simulink model "model_with_pursuit"  (R2023b)
settings: Solver=FixedStepAuto  StartTime=0.0  StopTime=10.0  FixedStep=Ts  RelTol=1e-3
values from neighbouring files (symbols this model uses):
  path = path * 0.1    [path_finder_waypoints.m]
  x0 = path(1,1)    [run_pp.m]
  y0 = path(1,2)    [run_pp.m]
undefined symbols (not defined in the file or in its folder): acceleration_limit, alpha, D, dist0, gear, J, Kb, Ki, Ki_turnrate, Kp, Kp_turnrate, Kt, L, M, R, taud, theta0, transport_delay, Ts, turn_acc_limit, wheel_distance, wrad, wzi
libraries: robotalgslib x1
settings Model: Creator=Gianluca  LastModifiedBy=simone

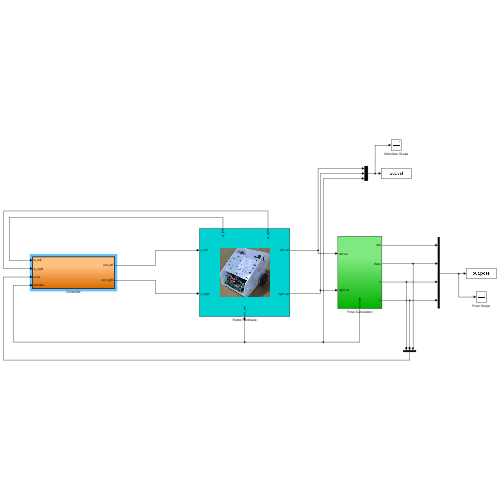
[thumbnail: Simulink's stored preview of the top-level diagram]
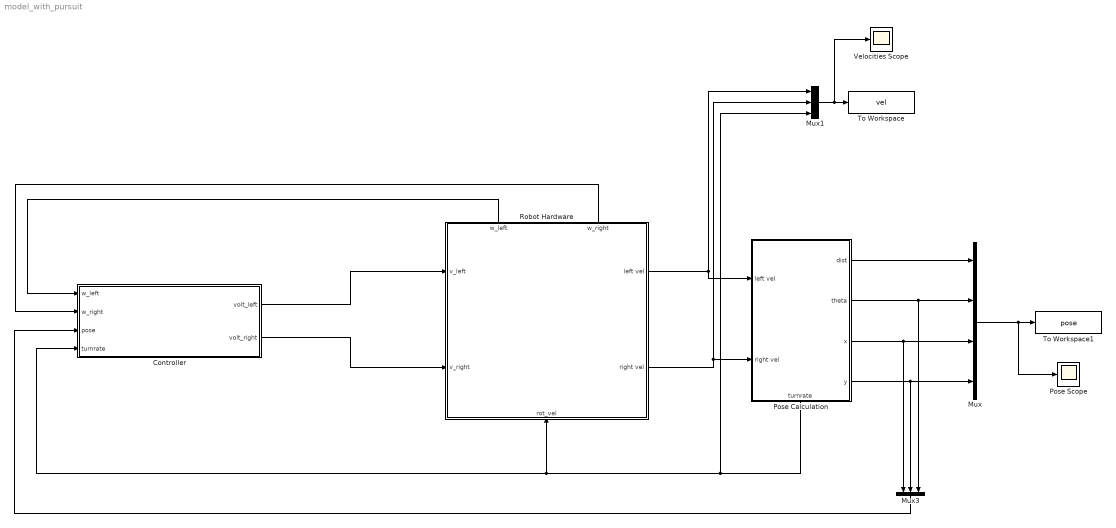
== system model_with_pursuit ==
  Controller : Subsystem  TreatAsAtomicUnit=on
  Mux : Mux
  Mux1 : Mux  Inputs=3
  Mux3 : Mux  Inputs=3
  Pose Calculation : Subsystem
      settings: PortSchema="{\"entries\":[{\"content\":{\"sides\":[{\"content\":{\"connectorIds\":[\"In1\",\"In2\"]},\"type\":\"ConnectorPlacement.EquallySpacedRectSide\",\"uuid\":\"46289eb4-3bbb-404a-99f0-e253fad6e87f\"},{\"content\":{\"connectorIds\":[\"Out1\",\"Out2\",\"Out3\",\"Out4\"],\"side\":\"RIGHT\"},\"type\":\"ConnectorPlacement.EquallySpacedRectSide\",\"uuid\":\"ccfc4e76-4e0e-4fcd-8da4-ce03e19c701c\"},{\"content\":{\"side\":\"TOP\"},\"type\":\"ConnectorPlacement.EquallySpacedRectSide\",\"uuid\":\"be5e5684-5a07-4d94-a4cd-7af4c2fd824b\"},{\"content\":{\"connectorIds\":[\"Out5\"],\"side\":\"BOTTOM\"},\"type\":\"ConnectorPlacement.EquallySpacedRectSide\",\"uuid\":\"5edce798-0d8e-42af-83a2-94dff7c31ae1\"}]},\"type\":\"ConnectorPlacement.EquallySpacedConnector\",\"uuid\":\"6a4a9bee-79c3-4932-b89c-a6fb8d0f2d92\"}],\"packageUris\":[\"http://schema.mathworks.com/mf0/Connector/R2020b\"],\"version\":\"1.0\"}"
  Pose Scope : Scope
  Robot Hardware : Subsystem
      settings: PortSchema="{\"entries\":[{\"content\":{\"sides\":[{\"content\":{\"connectorIds\":[\"In1\",\"In2\"]},\"type\":\"ConnectorPlacement.EquallySpacedRectSide\",\"uuid\":\"419fea77-f9ca-4e06-bea6-681a18650ab8\"},{\"content\":{\"connectorIds\":[\"Out1\",\"Out2\"],\"side\":\"RIGHT\"},\"type\":\"ConnectorPlacement.EquallySpacedRectSide\",\"uuid\":\"1629cad4-6101-470f-acc1-fad0cb327def\"},{\"content\":{\"connectorIds\":[\"Out3\",\"Out4\"],\"side\":\"TOP\"},\"type\":\"ConnectorPlacement.EquallySpacedRectSide\",\"uuid\":\"70c90e71-c188-4b9c-b220-781da08827f9\"},{\"content\":{\"connectorIds\":[\"In3\"],\"side\":\"BOTTOM\"},\"type\":\"ConnectorPlacement.EquallySpacedRectSide\",\"uuid\":\"9fee7d7d-5075-451a-8f6d-4cb9c8ead506\"}]},\"type\":\"ConnectorPlacement.EquallySpacedConnector\",\"uuid\":\"ad56978f-143c-418e-863d-6c6f1f6f5d0c\"}],\"packageUris\":[\"http://schema.mathworks.com/mf0/Connector/R2020b\"],\"version\":\"1.0\"}"
      mask Display: image('regbot.png');
  To Workspace : ToWorkspace  VariableName=vel  SaveFormat=Timeseries  SampleTime=-1
  To Workspace1 : ToWorkspace  VariableName=pose  SaveFormat=Timeseries  SampleTime=-1
  Velocities Scope : Scope
  wires:
  Pose Calculation/5(turnrate) -> Robot Hardware/3(rot_vel), Controller/4(turnrate), Mux1/3
  Robot Hardware/2(right vel) -> Mux1/2, Pose Calculation/2(right vel)
  Robot Hardware/1(left vel) -> Mux1/1, Pose Calculation/1(left vel)
  Mux/1 -> Pose Scope/1, To Workspace1/1
  Pose Calculation/2(theta) -> Mux/2, Mux3/3
  Pose Calculation/1(dist) -> Mux/1
  Mux1/1 -> Velocities Scope/1, To Workspace/1
  Pose Calculation/3(x) -> Mux/3, Mux3/1
  Pose Calculation/4(y) -> Mux3/2, Mux/4
  Robot Hardware/3(w_left) -> Controller/1(w_left)
  Robot Hardware/4(w_right) -> Controller/2(w_right)
  Mux3/1 -> Controller/3(pose)
  Controller/1(volt_left) -> Robot Hardware/1(v_left)
  Controller/2(volt_right) -> Robot Hardware/2(v_right)

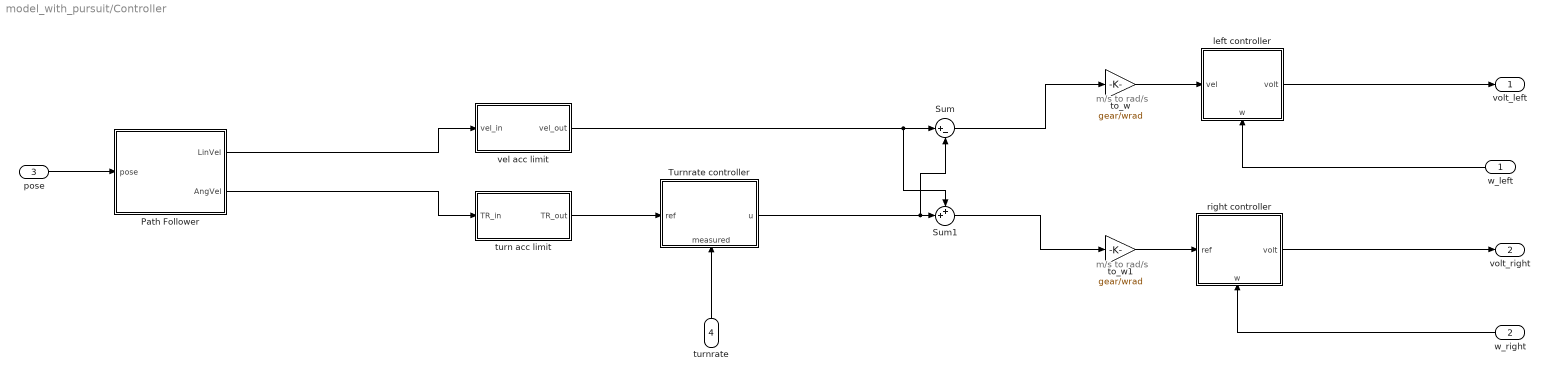
== system model_with_pursuit/Controller ==
  note: m/s to rad/s
  note: m/s to rad/s
  w_left : Inport
  w_right : Inport  Port=2
  pose : Inport  Port=3
  turnrate : Inport  Port=4
  Path Follower : Subsystem
  Sum : Sum  Inputs=|+-
  Sum1 : Sum  Inputs=++|
  Turnrate controller : Subsystem
      settings: PortSchema="{\"entries\":[{\"content\":{\"sides\":[{\"content\":{\"connectorIds\":[\"In1\"]},\"type\":\"ConnectorPlacement.EquallySpacedRectSide\",\"uuid\":\"3bde791d-a2ac-4d13-a51a-30874ee8f75a\"},{\"content\":{\"connectorIds\":[\"Out1\"],\"side\":\"RIGHT\"},\"type\":\"ConnectorPlacement.EquallySpacedRectSide\",\"uuid\":\"88ae4683-d3e7-483e-be55-3d26372f5fe2\"},{\"content\":{\"side\":\"TOP\"},\"type\":\"ConnectorPlacement.EquallySpacedRectSide\",\"uuid\":\"26752a72-f697-4de9-9dcd-1ca4cee0df39\"},{\"content\":{\"connectorIds\":[\"In2\"],\"side\":\"BOTTOM\"},\"type\":\"ConnectorPlacement.EquallySpacedRectSide\",\"uuid\":\"98a7b674-7c45-4a73-92a3-8750bdde1f36\"}]},\"type\":\"ConnectorPlacement.EquallySpacedConnector\",\"uuid\":\"d259c3e3-c5d7-42b6-881b-3a633aa969c6\"}],\"packageUris\":[\"http://schema.mathworks.com/mf0/Connector/R2020b\"],\"version\":\"1.0\"}"
  left controller : Subsystem
      settings: PortSchema="{\"entries\":[{\"content\":{\"sides\":[{\"content\":{\"connectorIds\":[\"In1\"]},\"type\":\"ConnectorPlacement.EquallySpacedRectSide\",\"uuid\":\"3bde791d-a2ac-4d13-a51a-30874ee8f75a\"},{\"content\":{\"connectorIds\":[\"Out1\"],\"side\":\"RIGHT\"},\"type\":\"ConnectorPlacement.EquallySpacedRectSide\",\"uuid\":\"88ae4683-d3e7-483e-be55-3d26372f5fe2\"},{\"content\":{\"side\":\"TOP\"},\"type\":\"ConnectorPlacement.EquallySpacedRectSide\",\"uuid\":\"26752a72-f697-4de9-9dcd-1ca4cee0df39\"},{\"content\":{\"connectorIds\":[\"In2\"],\"side\":\"BOTTOM\"},\"type\":\"ConnectorPlacement.EquallySpacedRectSide\",\"uuid\":\"8837b86a-35cd-4679-9975-e69b760c287c\"}]},\"type\":\"ConnectorPlacement.EquallySpacedConnector\",\"uuid\":\"d259c3e3-c5d7-42b6-881b-3a633aa969c6\"}],\"packageUris\":[\"http://schema.mathworks.com/mf0/Connector/R2020b\"],\"version\":\"1.0\"}"
  right controller : Subsystem
      settings: PortSchema="{\"entries\":[{\"content\":{\"sides\":[{\"content\":{\"connectorIds\":[\"In1\"]},\"type\":\"ConnectorPlacement.EquallySpacedRectSide\",\"uuid\":\"3bde791d-a2ac-4d13-a51a-30874ee8f75a\"},{\"content\":{\"connectorIds\":[\"Out1\"],\"side\":\"RIGHT\"},\"type\":\"ConnectorPlacement.EquallySpacedRectSide\",\"uuid\":\"88ae4683-d3e7-483e-be55-3d26372f5fe2\"},{\"content\":{\"side\":\"TOP\"},\"type\":\"ConnectorPlacement.EquallySpacedRectSide\",\"uuid\":\"26752a72-f697-4de9-9dcd-1ca4cee0df39\"},{\"content\":{\"connectorIds\":[\"In2\"],\"side\":\"BOTTOM\"},\"type\":\"ConnectorPlacement.EquallySpacedRectSide\",\"uuid\":\"1adabdfb-f360-4bb8-8b57-8160c74899b3\"}]},\"type\":\"ConnectorPlacement.EquallySpacedConnector\",\"uuid\":\"d259c3e3-c5d7-42b6-881b-3a633aa969c6\"}],\"packageUris\":[\"http://schema.mathworks.com/mf0/Connector/R2020b\"],\"version\":\"1.0\"}"
  to_w : Gain  Gain=gear/wrad
  to_w1 : Gain  Gain=gear/wrad
  turn acc limit : Subsystem
  vel acc limit : Subsystem
  volt_left : Outport
  volt_right : Outport  Port=2
  wires:
  Sum/1 -> to_w/1
  right controller/1(volt) -> volt_right/1
  Turnrate controller/1(u) -> Sum/2, Sum1/2
  left controller/1(volt) -> volt_left/1
  w_right/1 -> right controller/2(w)
  vel acc limit/1(vel_out) -> Sum1/1, Sum/1
  to_w1/1 -> right controller/1(ref)
  w_left/1 -> left controller/2(w)
  Sum1/1 -> to_w1/1
  turn acc limit/1(TR_out) -> Turnrate controller/1(ref)
  turnrate/1 -> Turnrate controller/2(measured)
  to_w/1 -> left controller/1(vel)
  Path Follower/1(LinVel) -> vel acc limit/1(vel_in)
  Path Follower/2(AngVel) -> turn acc limit/1(TR_in)
  pose/1 -> Path Follower/1(pose)

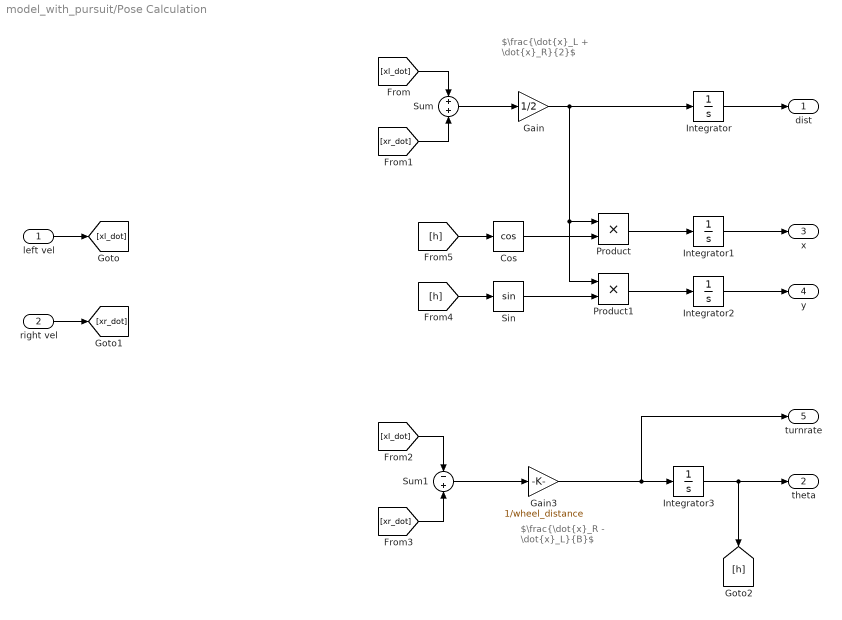
== system model_with_pursuit/Pose Calculation ==
  note: $\frac{\dot{x}_L + \dot{x}_R}{2}$
  note: $\frac{\dot{x}_R - \dot{x}_L}{B}$
  left vel : Inport
  right vel : Inport  Port=2
  Cos : Trigonometry  Operator=cos
  Gain : Gain  Gain=1/2
  Gain3 : Gain  Gain=1/wheel_distance
  Integrator : Integrator  InitialCondition=dist0
  Integrator1 : Integrator  InitialCondition=x0
  Integrator2 : Integrator  InitialCondition=y0
  Integrator3 : Integrator  InitialCondition=theta0
  Product : Product
  Product1 : Product
  Sin : Trigonometry
  Sum : Sum  Inputs=+|+
  Sum1 : Sum  Inputs=-|+
  dist : Outport
  theta : Outport  Port=2
  x : Outport  Port=3
  y : Outport  Port=4
  turnrate : Outport  Port=5
  wires:
  Sum/1 -> Gain/1
  Gain/1 -> Integrator/1, Product/1, Product1/1
  Integrator/1 -> dist/1
  left vel/1 -> [xl_dot]
  right vel/1 -> [xr_dot]
  [xl_dot] -> Sum/1
  [xr_dot] -> Sum/2
  [xl_dot] -> Sum1/1
  [xr_dot] -> Sum1/2
  Gain3/1 -> turnrate/1, Integrator3/1
  Sum1/1 -> Gain3/1
  Integrator3/1 -> theta/1, [h]
  [h] -> Sin/1
  Integrator2/1 -> y/1
  Integrator1/1 -> x/1
  [h] -> Cos/1
  Sin/1 -> Product1/2
  Cos/1 -> Product/2
  Product1/1 -> Integrator2/1
  Product/1 -> Integrator1/1

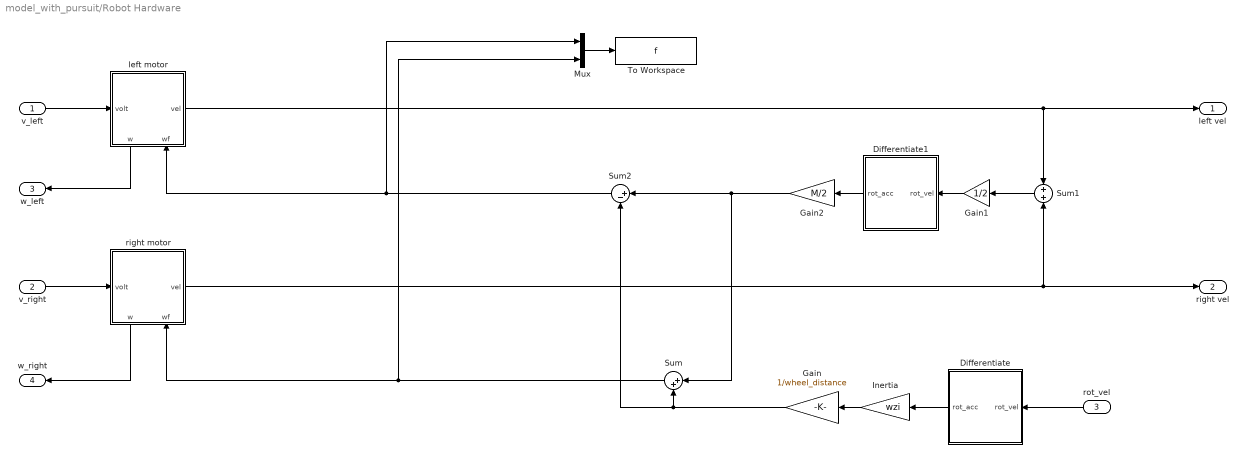
== system model_with_pursuit/Robot Hardware ==
  v_left : Inport
  v_right : Inport  Port=2
  rot_vel : Inport  Port=3
  Differentiate : Subsystem
  Differentiate1 : Subsystem
  Gain : Gain  Gain=1/wheel_distance
  Gain1 : Gain  Gain=1/2
  Gain2 : Gain  Gain=M/2
  Inertia : Gain  Gain=wzi
  Mux : Mux  Inputs=2
  Sum : Sum  Inputs=|++
  Sum1 : Sum  Inputs=+|+
  Sum2 : Sum  Inputs=|+-
  To Workspace : ToWorkspace  VariableName=f  SaveFormat=Timeseries  SampleTime=-1
  left motor : Subsystem
      settings: PortSchema="{\"entries\":[{\"content\":{\"sides\":[{\"content\":{\"connectorIds\":[\"In1\"]},\"type\":\"ConnectorPlacement.EquallySpacedRectSide\",\"uuid\":\"3bde791d-a2ac-4d13-a51a-30874ee8f75a\"},{\"content\":{\"connectorIds\":[\"Out1\"],\"side\":\"RIGHT\"},\"type\":\"ConnectorPlacement.EquallySpacedRectSide\",\"uuid\":\"88ae4683-d3e7-483e-be55-3d26372f5fe2\"},{\"content\":{\"side\":\"TOP\"},\"type\":\"ConnectorPlacement.EquallySpacedRectSide\",\"uuid\":\"26752a72-f697-4de9-9dcd-1ca4cee0df39\"},{\"content\":{\"connectorIds\":[\"Out2\",\"In2\"],\"side\":\"BOTTOM\"},\"type\":\"ConnectorPlacement.EquallySpacedRectSide\",\"uuid\":\"bdf58d17-97a4-48aa-9393-076eaaeca649\"}]},\"type\":\"ConnectorPlacement.EquallySpacedConnector\",\"uuid\":\"d259c3e3-c5d7-42b6-881b-3a633aa969c6\"}],\"packageUris\":[\"http://schema.mathworks.com/mf0/Connector/R2020b\"],\"version\":\"1.0\"}"
  right motor : Subsystem
      settings: PortSchema="{\"entries\":[{\"content\":{\"sides\":[{\"content\":{\"connectorIds\":[\"In1\"]},\"type\":\"ConnectorPlacement.EquallySpacedRectSide\",\"uuid\":\"3bde791d-a2ac-4d13-a51a-30874ee8f75a\"},{\"content\":{\"connectorIds\":[\"Out1\"],\"side\":\"RIGHT\"},\"type\":\"ConnectorPlacement.EquallySpacedRectSide\",\"uuid\":\"88ae4683-d3e7-483e-be55-3d26372f5fe2\"},{\"content\":{\"side\":\"TOP\"},\"type\":\"ConnectorPlacement.EquallySpacedRectSide\",\"uuid\":\"26752a72-f697-4de9-9dcd-1ca4cee0df39\"},{\"content\":{\"connectorIds\":[\"Out2\",\"In2\"],\"side\":\"BOTTOM\"},\"type\":\"ConnectorPlacement.EquallySpacedRectSide\",\"uuid\":\"bdf58d17-97a4-48aa-9393-076eaaeca649\"}]},\"type\":\"ConnectorPlacement.EquallySpacedConnector\",\"uuid\":\"d259c3e3-c5d7-42b6-881b-3a633aa969c6\"}],\"packageUris\":[\"http://schema.mathworks.com/mf0/Connector/R2020b\"],\"version\":\"1.0\"}"
  left vel : Outport
  right vel : Outport  Port=2
  w_left : Outport  Port=3
  w_right : Outport  Port=4
  wires:
  v_left/1 -> left motor/1(volt)
  left motor/2(w) -> w_left/1
  v_right/1 -> right motor/1(volt)
  right motor/2(w) -> w_right/1
  Mux/1 -> To Workspace/1
  rot_vel/1 -> Differentiate/1(rot_vel)
  Differentiate/1(rot_acc) -> Inertia/1
  Inertia/1 -> Gain/1
  Gain/1 -> Sum/2, Sum2/2
  Sum/1 -> right motor/2(wf), Mux/2
  left motor/1(vel) -> Sum1/1, left vel/1
  Sum1/1 -> Gain1/1
  Gain1/1 -> Differentiate1/1(rot_vel)
  Differentiate1/1(rot_acc) -> Gain2/1
  Gain2/1 -> Sum/1, Sum2/1
  Sum2/1 -> left motor/2(wf), Mux/1
  right motor/1(vel) -> Sum1/2, right vel/1

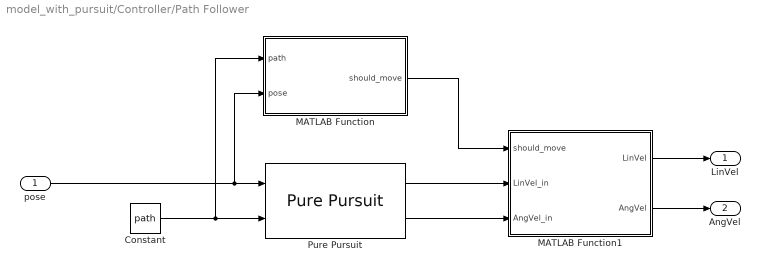
== system model_with_pursuit/Controller/Path Follower ==
  pose : Inport
  Constant : Constant  Value=path
  MATLAB Function : MATLAB Function  TreatAsAtomicUnit=on
  MATLAB Function1 : MATLAB Function  TreatAsAtomicUnit=on
  Pure Pursuit : robotalgslib/Pure Pursuit  DesiredLinearVelocity=vel_ref  MaxAngularVelocity=turn_acc_limit  LookaheadDistance=lookahead_dist  TargetDirPort=off  SimulateUsing=Code generation
      settings: LibrarySourceBlock=navlib/Control Algorithms/Pure Pursuit
  LinVel : Outport
  AngVel : Outport  Port=2
  wires:
  MATLAB Function/1(should_move) -> MATLAB Function1/1(should_move)
  pose/1 -> MATLAB Function/2(pose), Pure Pursuit/1
  MATLAB Function1/1(LinVel) -> LinVel/1
  MATLAB Function1/2(AngVel) -> AngVel/1
  Pure Pursuit/1 -> MATLAB Function1/2(LinVel_in)
  Pure Pursuit/2 -> MATLAB Function1/3(AngVel_in)
  Constant/1 -> MATLAB Function/1(path), Pure Pursuit/2

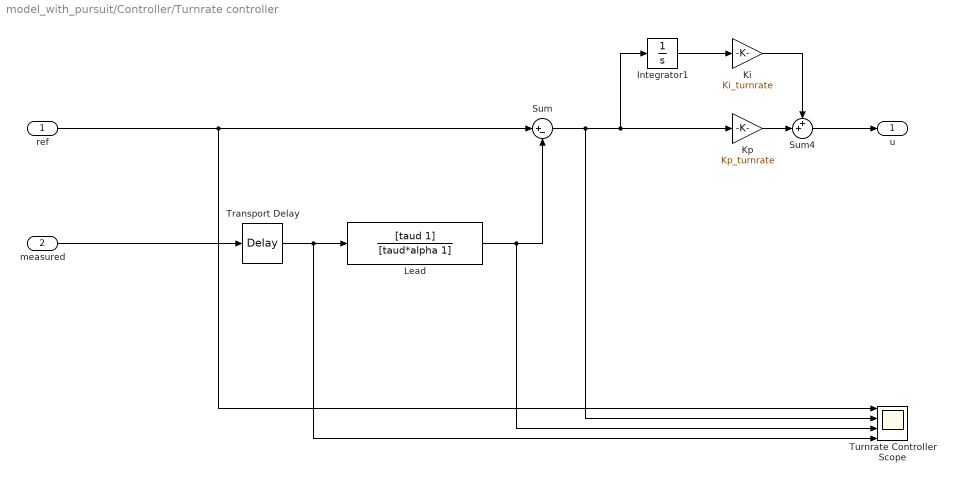
== system model_with_pursuit/Controller/Turnrate controller ==
  ref : Inport
  measured : Inport  Port=2
  Integrator1 : Integrator
  Ki : Gain  Gain=Ki_turnrate
  Kp : Gain  Gain=Kp_turnrate
  Lead : TransferFcn  Numerator=[taud 1]  Denominator=[taud*alpha 1]
  Sum : Sum  Inputs=|+-
  Sum4 : Sum  Inputs=++|
  Transport Delay : TransportDelay  DelayTime=transport_delay
  Turnrate Controller Scope : Scope  NumInputPorts=4
  u : Outport
  wires:
  ref/1 -> Turnrate Controller Scope/1, Sum/1
  Lead/1 -> Sum/2, Turnrate Controller Scope/3
  measured/1 -> Transport Delay/1
  Transport Delay/1 -> Turnrate Controller Scope/4, Lead/1
  Sum4/1 -> u/1
  Sum/1 -> Turnrate Controller Scope/2, Integrator1/1, Kp/1
  Integrator1/1 -> Ki/1
  Ki/1 -> Sum4/1
  Kp/1 -> Sum4/2

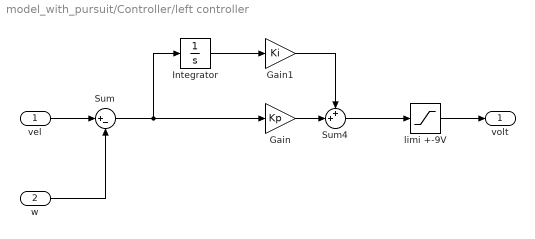
== system model_with_pursuit/Controller/left controller ==
  vel : Inport
  w : Inport  Port=2
  Gain : Gain  Gain=Kp
  Gain1 : Gain  Gain=Ki
  Integrator : Integrator
  Sum : Sum  Inputs=|+-
  Sum4 : Sum  Inputs=++|
  limi +-9V : Saturate  UpperLimit=9  LowerLimit=-9
  volt : Outport
  wires:
  Gain/1 -> Sum4/2
  Integrator/1 -> Gain1/1
  Gain1/1 -> Sum4/1
  vel/1 -> Sum/1
  w/1 -> Sum/2
  Sum/1 -> Integrator/1, Gain/1
  Sum4/1 -> limi +-9V/1
  limi +-9V/1 -> volt/1

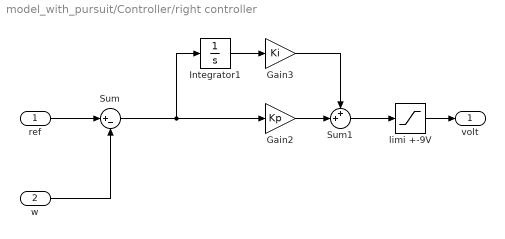
== system model_with_pursuit/Controller/right controller ==
  ref : Inport
  w : Inport  Port=2
  Gain2 : Gain  Gain=Kp
  Gain3 : Gain  Gain=Ki
  Integrator1 : Integrator
  Sum : Sum  Inputs=|+-
  Sum1 : Sum  Inputs=++|
  limi +-9V : Saturate  UpperLimit=9  LowerLimit=-9
  volt : Outport
  wires:
  Integrator1/1 -> Gain3/1
  Gain2/1 -> Sum1/2
  Gain3/1 -> Sum1/1
  Sum/1 -> Integrator1/1, Gain2/1
  ref/1 -> Sum/1
  w/1 -> Sum/2
  Sum1/1 -> limi +-9V/1
  limi +-9V/1 -> volt/1

== system model_with_pursuit/Controller/turn acc limit ==
  TR_in : Inport
  Gain : Gain  Gain=100
  Integrator : Integrator
  Saturation : Saturate  UpperLimit=turn_acc_limit  LowerLimit=-turn_acc_limit
  Sum : Sum  Inputs=|+-
  TR_out : Outport
  wires:
  TR_in/1 -> Sum/1
  Sum/1 -> Gain/1
  Gain/1 -> Saturation/1
  Saturation/1 -> Integrator/1
  Integrator/1 -> Sum/2, TR_out/1

== system model_with_pursuit/Controller/vel acc limit ==
  vel_in : Inport
  Gain : Gain  Gain=100
  Integrator : Integrator
  Saturation : Saturate  UpperLimit=acceleration_limit  LowerLimit=-acceleration_limit
  Sum : Sum  Inputs=|+-
  vel_out : Outport
  wires:
  vel_in/1 -> Sum/1
  Sum/1 -> Gain/1
  Gain/1 -> Saturation/1
  Saturation/1 -> Integrator/1
  Integrator/1 -> Sum/2, vel_out/1

== system model_with_pursuit/Robot Hardware/Differentiate ==
  rot_vel : Inport
  Gain : Gain  Gain=100
  Integrator : Integrator
  Sum : Sum  Inputs=|+-
  rot_acc : Outport
  wires:
  rot_vel/1 -> Sum/1
  Sum/1 -> Gain/1
  Integrator/1 -> Sum/2
  Gain/1 -> rot_acc/1, Integrator/1

== system model_with_pursuit/Robot Hardware/Differentiate1 ==
  rot_vel : Inport
  Gain : Gain  Gain=100
  Integrator : Integrator
  Sum : Sum  Inputs=|+-
  rot_acc : Outport
  wires:
  rot_vel/1 -> Sum/1
  Sum/1 -> Gain/1
  Integrator/1 -> Sum/2
  Gain/1 -> rot_acc/1, Integrator/1

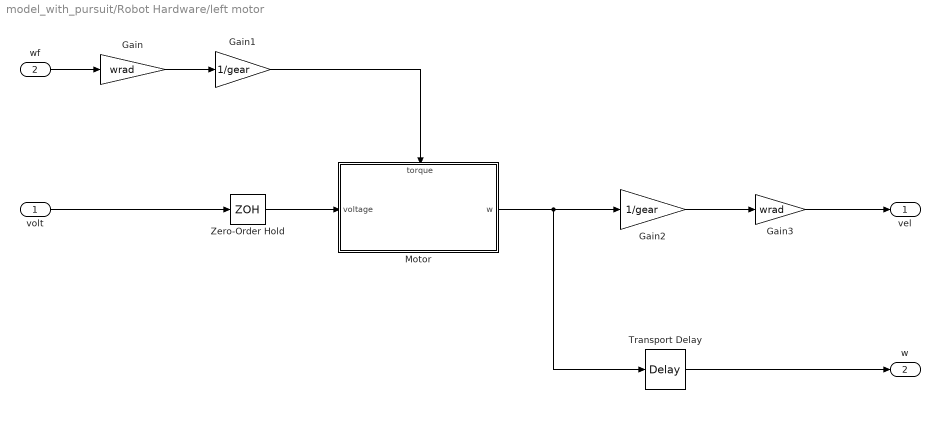
== system model_with_pursuit/Robot Hardware/left motor ==
  volt : Inport
  wf : Inport  Port=2
  Gain : Gain  Gain=wrad
  Gain1 : Gain  Gain=1/gear
  Gain2 : Gain  Gain=1/gear
  Gain3 : Gain  Gain=wrad
  Motor : Subsystem
      settings: PortSchema="{\"entries\":[{\"content\":{\"sides\":[{\"content\":{\"connectorIds\":[\"In1\"]},\"type\":\"ConnectorPlacement.EquallySpacedRectSide\",\"uuid\":\"3bde791d-a2ac-4d13-a51a-30874ee8f75a\"},{\"content\":{\"connectorIds\":[\"Out1\"],\"side\":\"RIGHT\"},\"type\":\"ConnectorPlacement.EquallySpacedRectSide\",\"uuid\":\"88ae4683-d3e7-483e-be55-3d26372f5fe2\"},{\"content\":{\"connectorIds\":[\"In2\"],\"side\":\"TOP\"},\"type\":\"ConnectorPlacement.EquallySpacedRectSide\",\"uuid\":\"26752a72-f697-4de9-9dcd-1ca4cee0df39\"}]},\"type\":\"ConnectorPlacement.EquallySpacedConnector\",\"uuid\":\"d259c3e3-c5d7-42b6-881b-3a633aa969c6\"}],\"packageUris\":[\"http://schema.mathworks.com/mf0/Connector/R2020b\"],\"version\":\"1.0\"}"
  Transport Delay : TransportDelay  DelayTime=transport_delay
  Zero-Order Hold : ZeroOrderHold  SampleTime=Ts
  vel : Outport
  w : Outport  Port=2
  wires:
  wf/1 -> Gain/1
  Gain/1 -> Gain1/1
  Gain1/1 -> Motor/2(torque)
  Gain3/1 -> vel/1
  Gain2/1 -> Gain3/1
  Motor/1(w) -> Transport Delay/1, Gain2/1
  Transport Delay/1 -> w/1
  volt/1 -> Zero-Order Hold/1
  Zero-Order Hold/1 -> Motor/1(voltage)

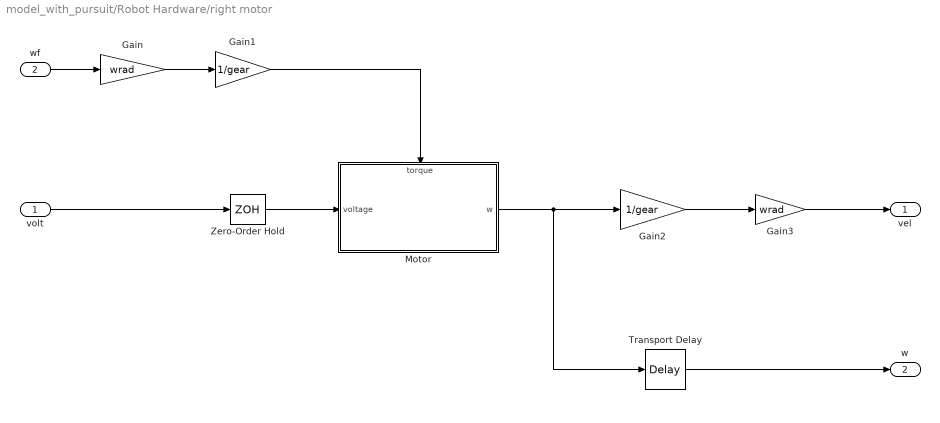
== system model_with_pursuit/Robot Hardware/right motor ==
  volt : Inport
  wf : Inport  Port=2
  Gain : Gain  Gain=wrad
  Gain1 : Gain  Gain=1/gear
  Gain2 : Gain  Gain=1/gear
  Gain3 : Gain  Gain=wrad
  Motor : Subsystem
      settings: PortSchema="{\"entries\":[{\"content\":{\"sides\":[{\"content\":{\"connectorIds\":[\"In1\"]},\"type\":\"ConnectorPlacement.EquallySpacedRectSide\",\"uuid\":\"3bde791d-a2ac-4d13-a51a-30874ee8f75a\"},{\"content\":{\"connectorIds\":[\"Out1\"],\"side\":\"RIGHT\"},\"type\":\"ConnectorPlacement.EquallySpacedRectSide\",\"uuid\":\"88ae4683-d3e7-483e-be55-3d26372f5fe2\"},{\"content\":{\"connectorIds\":[\"In2\"],\"side\":\"TOP\"},\"type\":\"ConnectorPlacement.EquallySpacedRectSide\",\"uuid\":\"26752a72-f697-4de9-9dcd-1ca4cee0df39\"}]},\"type\":\"ConnectorPlacement.EquallySpacedConnector\",\"uuid\":\"d259c3e3-c5d7-42b6-881b-3a633aa969c6\"}],\"packageUris\":[\"http://schema.mathworks.com/mf0/Connector/R2020b\"],\"version\":\"1.0\"}"
  Transport Delay : TransportDelay  DelayTime=transport_delay
  Zero-Order Hold : ZeroOrderHold  SampleTime=Ts
  vel : Outport
  w : Outport  Port=2
  wires:
  wf/1 -> Gain/1
  Gain/1 -> Gain1/1
  Gain1/1 -> Motor/2(torque)
  Gain3/1 -> vel/1
  Gain2/1 -> Gain3/1
  Motor/1(w) -> Transport Delay/1, Gain2/1
  Transport Delay/1 -> w/1
  volt/1 -> Zero-Order Hold/1
  Zero-Order Hold/1 -> Motor/1(voltage)

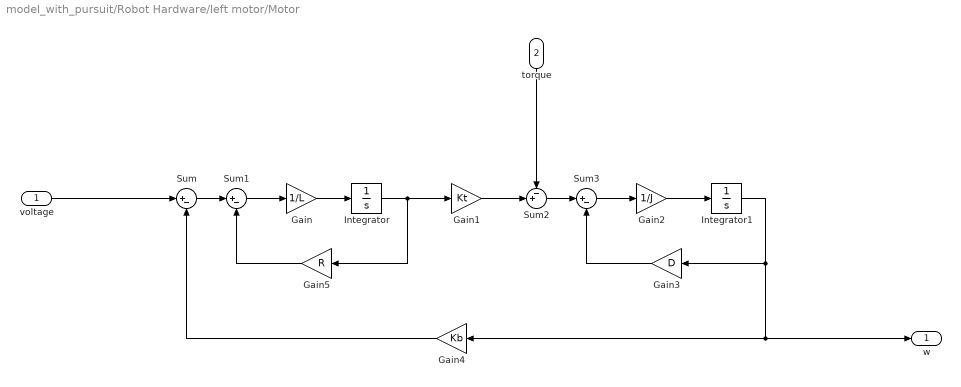
== system model_with_pursuit/Robot Hardware/left motor/Motor ==
  voltage : Inport
  torque : Inport  Port=2
  Gain : Gain  Gain=1/L
  Gain1 : Gain  Gain=Kt
  Gain2 : Gain  Gain=1/J
  Gain3 : Gain  Gain=D
  Gain4 : Gain  Gain=Kb
  Gain5 : Gain  Gain=R
  Integrator : Integrator
  Integrator1 : Integrator
  Sum : Sum  Inputs=|+-
  Sum1 : Sum  Inputs=|+-
  Sum2 : Sum  Inputs=-+|
  Sum3 : Sum  Inputs=|+-
  w : Outport
  wires:
  voltage/1 -> Sum/1
  Sum/1 -> Sum1/1
  Gain/1 -> Integrator/1
  Gain1/1 -> Sum2/2
  Integrator/1 -> Gain5/1, Gain1/1
  torque/1 -> Sum2/1
  Sum2/1 -> Sum3/1
  Sum3/1 -> Gain2/1
  Gain2/1 -> Integrator1/1
  Integrator1/1 -> Gain3/1, Gain4/1, w/1
  Gain3/1 -> Sum3/2
  Gain4/1 -> Sum/2
  Gain5/1 -> Sum1/2
  Sum1/1 -> Gain/1

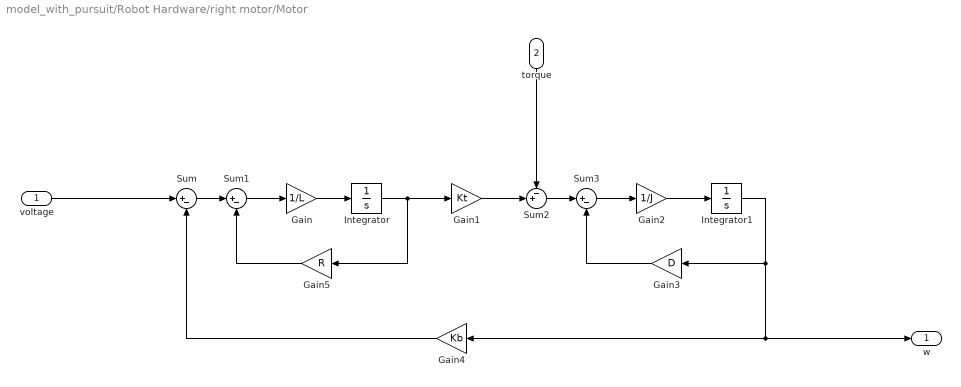
== system model_with_pursuit/Robot Hardware/right motor/Motor ==
  voltage : Inport
  torque : Inport  Port=2
  Gain : Gain  Gain=1/L
  Gain1 : Gain  Gain=Kt
  Gain2 : Gain  Gain=1/J
  Gain3 : Gain  Gain=D
  Gain4 : Gain  Gain=Kb
  Gain5 : Gain  Gain=R
  Integrator : Integrator
  Integrator1 : Integrator
  Sum : Sum  Inputs=|+-
  Sum1 : Sum  Inputs=|+-
  Sum2 : Sum  Inputs=-+|
  Sum3 : Sum  Inputs=|+-
  w : Outport
  wires:
  voltage/1 -> Sum/1
  Sum/1 -> Sum1/1
  Gain/1 -> Integrator/1
  Gain1/1 -> Sum2/2
  Integrator/1 -> Gain5/1, Gain1/1
  torque/1 -> Sum2/1
  Sum2/1 -> Sum3/1
  Sum3/1 -> Gain2/1
  Gain2/1 -> Integrator1/1
  Integrator1/1 -> Gain3/1, Gain4/1, w/1
  Gain3/1 -> Sum3/2
  Gain4/1 -> Sum/2
  Gain5/1 -> Sum1/2
  Sum1/1 -> Gain/1

== matlab function model_with_pursuit/Controller/Path Follower/MATLAB Function1 ==
  data: should_move input; LinVel output; LinVel_in input; AngVel_in input; AngVel output
function [LinVel, AngVel] = get_res(should_move, LinVel_in, AngVel_in)

if should_move
    LinVel = LinVel_in;
    AngVel = AngVel_in;
else
    LinVel = 0;
    AngVel = 0;
end

== matlab function model_with_pursuit/Controller/Path Follower/MATLAB Function ==
  data: path input; should_move output; pose input
function should_move = are_we_at_goal(path, pose)

pose = pose([1 2], :)';
robotGoal = path(end, :);

goalRadius = 0.05;
distanceToGoal = norm(pose - robotGoal);

if distanceToGoal < goalRadius
    should_move = 0;
else
    should_move = 1;
end
